simulink model "IP_LQR"  (R2020b)
settings: Solver=VariableStepAuto  StartTime=0.0  StopTime=5  RelTol=1e-3
values from neighbouring files (symbols this model uses):
  A = [0       1              0         0 ... (first row only)    [IP_Design.m]
  B = [     0 ... (first row only)    [IP_Design.m]
  C = [1 0 0 0 ... (first row only)    [IP_Design.m]
  D = zeros(2,1)    [IP_Design.m]
  K = lqr(A,B,Q,R)    [IP_Design.m]
  L = place(A',C',P)'    [IP_Design.m]
  m = 0.2    [Data_for_IP_Sim_Model.m]    (also in IP_Design.m)
  N = -1/(C*inv(Ac)*B)    [IP_Design.m]
  Qk = 0.005    [IP_Design.m]
  Rk = 0.001    [IP_Design.m]
  Sf = N(1,1)    [IP_Design.m]
undefined symbols (not defined in the file or in its folder): Continuous, sigbuilder_block, Time, X, Y, Z
libraries: sm_lib x8, nesl_utility x6, ctrlSharedLib x1
settings Model: Creator=tushark  LastModifiedBy=raghavendrans
settings ExplorerConfigSet: InternalSimMechanicsExplorerSettings="<ExplorerConfiguration><canonicalview>default</canonicalview><AnimationSetting><BasePlaybackSpeed>1.0</BasePlaybackSpeed><PlaybackSpeedFactor>1.0</PlaybackSpeedFactor></AnimationSetting><TilePanel><TileInfo><Tiles Columns=\"1\" Count=\"1\" Rows=\"1\"><Column Weight=\"1\"/><Row Weight=\"1\"/><Tile Height=\"1\" Width=\"1\" X=\"0\" Y=\"0\"/></Tiles></TileInfo><SceneInfo><SceneViewer><BGColor><R>1</R><G>1</G><B>1</B></BGColor><Camera><DoPerspective>off</DoPerspective><Position><X>0.288705906044352034</X><Y>-0.999999988114421923</Y><Z>0.250006416228108375</Z></Position><Center><X>0.288705906044352034</X><Y>1.18855781328086607e-08</Y><Z>0.250006416228108375</Z></Center><Up><X>0</X><Y>-0</Y><Z>1</Z></Up><ViewLimDist>1</ViewLimDist><YLim>0.360506624281406396</YLim><XLim>0.67276188393623837</XLim></Camera></SceneViewer></SceneInfo></TilePanel><MechEditorPanel><Cameras/><GfxPanelCameraMap/><VideoCreator><PlaybackSpeedRatio>1.0</PlaybackSpeedRatio><FrameRate>30</FrameRate><VideoFormat>Motion JPEG AVI</VideoFormat><FrameSize>auto</FrameSize></VideoCreator></MechEditorPanel></ExplorerConfiguration>"

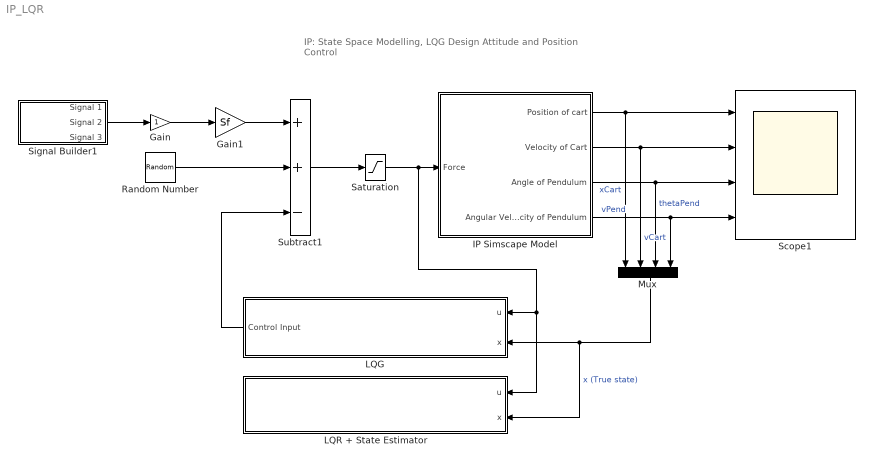
== system IP_LQR ==
  note: IP: State Space Modelling, LQG Design
      | Attitude and Position Control
  Gain : Gain
  Gain1 : Gain  Gain=Sf
  IP Simscape Model : Subsystem
  LQG : Subsystem
  LQR + State Estimator : Subsystem
  Mux : Mux
  Random Number : RandomNumber  Variance=Qk  SampleTime=0.1
  Saturation : Saturate  UpperLimit=1  LowerLimit=-1
  Scope1 : Scope  NumInputPorts=4
  Signal Builder1 : Subsystem  Tag=STV Subsys  LoadFcn=sigbuilder_block('load');  StartFcn=sigbuilder_block('start');  StopFcn=sigbuilder_block('stop');  ClipboardFcn=sigbuilder_block('clipboard');  mask(Sigbuilder block){tuvar=[0:10]}
      mask help: Simulink:masks:SigbuilderBlock_MD
      mask init:
      | if ~strcmp(get_param(bdroot(gcbh),'SimulationStatus'),'stopped') tuvar = sigbuilder_block('maskInit'); end
      settings: CopyFcn=sigbuilder_block('copy');  DeleteFcn=sigbuilder_block('delete');  ModelCloseFcn=sigbuilder_block('modelClose');  PreSaveFcn=sigbuilder_block('preSave');  PauseFcn=sigbuilder_block('pause');  ContinueFcn=sigbuilder_block('continue');  NameChangeFcn=sigbuilder_block('namechange');  OpenFcn=sigbuilder_block('open',[437.6 199.2 550.4 400 ]);  CloseFcn=sigbuilder_block('close');
      mask Display: plot(0, 0, 100, 100,[2, 2, 32, 32, 2], [68, 8, 8, 68, 68],[32, 2], [38, 38], [32, 19, 2],[53, 60, 44], [32, 17, 17, 2],[16, 16, 31, 31]);txt = getActiveGroup(gcbh);text(2, 100, txt,'verticalAlignment', 'top');
  Subtract1 : Sum  Inputs=++-
  wires:
  IP Simscape Model/1(Position of cart) -> Scope1/1, Mux/1  "xCart"
  IP Simscape Model/4(Angular Velocity of Pendulum) -> Scope1/4, Mux/4  "vPend"
  IP Simscape Model/3(Angle of Pendulum) -> Scope1/3, Mux/3  "thetaPend"
  IP Simscape Model/2(Velocity of Cart) -> Scope1/2, Mux/2  "vCart"
  Gain1/1 -> Subtract1/1
  Saturation/1 -> IP Simscape Model/1("Force "), LQR + State Estimator/1(u), LQG/1(u)
  Subtract1/1 -> Saturation/1
  Mux/1 -> LQR + State Estimator/2(x), LQG/2(x)  "x (True state)"
  Gain/1 -> Gain1/1
  Signal Builder1/2(Signal 2) -> Gain/1
  Random Number/1 -> Subtract1/2
  LQG/1("Control Input ") -> Subtract1/3

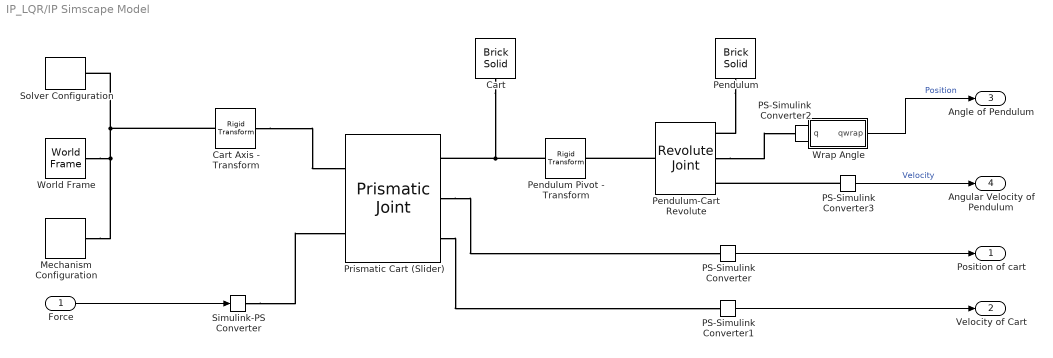
== system IP_LQR/IP Simscape Model ==
  "Force " : Inport
  Cart : sm_lib/Body Elements/Brick Solid  GraphicAmbientColor=[0.15 0.15 0.15 1.0]  BasedOnType=Density  BrickDimensions=[0.2 0.04 0.6]  BrickDimensionUnits=m  CenterOfMass=[0 0 0]  CenterOfMassUnits=m  GraphicDiffuseColor=[1.0 0.2 0.2]  Density=1000  DensityUnits=kg/m^3  DoExposeReferenceFrame=on  GraphicEmissiveColor=[0.0 0.0 0.0 1.0]  ExportEntireGeometry=off  SerializedFrames=<Frames/>  MarkerShape=Sphere  MarkerSize=10  GraphicType=FromGeometry  InertiaType=PointMass  Mass=0.5  MassUnits=kg  MomentsOfInertia=[1 1 1]  MomentsOfInertiaUnits=kg*m^2  GraphicOpacity=1.0  ProductsOfInertia=[0 0 0]  ProductsOfInertiaUnits=kg*m^2  GraphicShininess=75  GraphicSpecularColor=[0.5 0.5 0.5 1.0]  GraphicVisPropType=SimpleVisualProperties
  Cart Axis - Transform : sm_lib/Frames and Transforms/Rigid Transform  TranslationMethod=None  TranslationStandardOffset=0  TranslationLengthUnit=m  TranslationStandardAxis=+Z  TranslationCartesianOffset=[0 0 0]  TranslationROffset=0  TranslationROffsetUnits=m  TranslationZOffset=0  TranslationZOffsetUnits=m  TranslationThetaOffset=0  TranslationThetaOffsetUnits=deg  RotationMethod=StandardAxis  RotationAngleUnits=deg  RotationStandardAxis=+Y  RotationAngle=90  RotationArbitraryAxis=[0 0 1]  FollAlignAxisA=+X  BaseAlignAxisA=+Y  FollAlignAxisB=+Y  BaseAlignAxisB=+Z  RotationSequenceAxes=FollowerAxes  RotationSequence=XYX  RotationSequenceAngles=[0 0 0]  RotationSequenceAnglesUnits=deg  RotationMatrix=[1 0 0; 0 1 0; 0 0 1]
      settings: SourceProductName=Multibody
  Mechanism Configuration : sm_lib/Utilities/Mechanism Configuration  UniformGravity=Constant  GravityVector=[0 0 -9.80665]  GravityVectorUnits=m/s^2  GravityUnits=m/s^2  LinearizationDelta=0.001  JointModeTransitionNonlinearIterations=2
      settings: SourceProductName=Multibody
  PS-Simulink Converter{,1..3} (4 alike) : nesl_utility/PS-Simulink Converter  PhysicalDomain=network_engine_domain  SubClassName=ps_output  LeftPortType=input  RightPortType=output  PseudoPeriodic=off  Frequencies=[]  Unit=inherit  AffineConversion=off
  Pendulum : sm_lib/Body Elements/Brick Solid  GraphicAmbientColor=[0.15 0.15 0.15 1.0]  BasedOnType=Density  BrickDimensions=[0.6 0.03 0.05]  BrickDimensionUnits=m  CenterOfMass=[0 0 0]  CenterOfMassUnits=m  GraphicDiffuseColor=[0.0 0.4 1.0]  Density=1000  DensityUnits=kg/m^3  DoExposeReferenceFrame=off  GraphicEmissiveColor=[0.0 0.0 0.0 1.0]  ExportEntireGeometry=off  SerializedFrames=<Frames><Frame><Id>Frame1</Id><Value><Name>P</Name><Origin><Source>GeometricFeature</Source><FeatureName>+x surface</FeatureName></Origin><PrimaryAxis><DefinedDirection>+Z</DefinedDirection><Source>ReferenceFrame</Source><SourceDirection>+Z</SourceDirection><FeatureName></FeatureName></PrimaryAxis><SecondaryAxis><DefinedDirection>+X</DefinedDirection><Source>ReferenceFrame</Source><SourceDirection>+X</SourceDirection><FeatureName></FeatureName></SecondaryAxis></Value></Frame></Frames>  MarkerShape=Sphere  MarkerSize=10  GraphicType=FromGeometry  InertiaType=PointMass  Mass=0.2  MassUnits=kg  MomentsOfInertia=[1 1 1]  MomentsOfInertiaUnits=kg*m^2  GraphicOpacity=1.0  ProductsOfInertia=[0 0 0]  ProductsOfInertiaUnits=kg*m^2  GraphicShininess=75  GraphicSpecularColor=[0.5 0.5 0.5 1.0]  GraphicVisPropType=SimpleVisualProperties
  Pendulum Pivot - Transform : sm_lib/Frames and Transforms/Rigid Transform  TranslationMethod=None  TranslationStandardOffset=0  TranslationLengthUnit=m  TranslationStandardAxis=+Z  TranslationCartesianOffset=[0 0 0]  TranslationROffset=0  TranslationROffsetUnits=m  TranslationZOffset=0  TranslationZOffsetUnits=m  TranslationThetaOffset=0  TranslationThetaOffsetUnits=deg  RotationMethod=StandardAxis  RotationAngleUnits=deg  RotationStandardAxis=+X  RotationAngle=90  RotationArbitraryAxis=[0 0 1]  FollAlignAxisA=+X  BaseAlignAxisA=+Y  FollAlignAxisB=+Y  BaseAlignAxisB=+Z  RotationSequenceAxes=FollowerAxes  RotationSequence=XYX  RotationSequenceAngles=[0 0 0]  RotationSequenceAnglesUnits=deg  RotationMatrix=[1 0 0; 0 1 0; 0 0 1]
      settings: SourceProductName=Multibody
  Pendulum-Cart Revolute : sm_lib/Joints/Revolute Joint  JointMode=Normal  SenseConstraintForce=off  SenseConstraintForceX=off  SenseConstraintForceY=off  SenseConstraintForceZ=off  SenseConstraintTorque=off  SenseConstraintTorqueX=off  SenseConstraintTorqueY=off  SenseConstraintTorqueZ=off  SenseTotalForce=off  SenseTotalForceX=off  SenseTotalForceY=off  SenseTotalForceZ=off  SenseTotalTorque=off  SenseTotalTorqueX=off  SenseTotalTorqueY=off  SenseTotalTorqueZ=off  CompositeWrenchDir=FollowerOnBase  CompositeWrenchFrame=BaseFrame  EquilibriumPosition=0  EquilibriumPositionUnits=deg  SpringStiffness=0  SpringStiffnessUnits=N*m/deg  DampingCoefficient=0  DampingCoefficientUnits=N*m/(deg/s)  TorqueActuationMode=NoTorque  MotionActuationMode=ComputedMotion  SensePosition=on  SenseVelocity=on  SenseAcceleration=off  SenseTorqueForce=off  SenseLowerLimitTorqueForce=off  SenseUpperLimitTorqueForce=off  LowerLimitSpecify=off  LowerLimitBound=-90  LowerLimitBoundUnits=deg  LowerLimitStiffness=1e4  LowerLimitStiffnessUnits=N*m/deg  LowerLimitDamping=10  LowerLimitDampingUnits=N*m/(deg/s)  LowerLimitTransitionRegionWidth=0.1  LowerLimitTransitionRegionWidthUnits=deg  UpperLimitSpecify=off  UpperLimitBound=90  UpperLimitBoundUnits=deg  UpperLimitStiffness=1e4  UpperLimitStiffnessUnits=N*m/deg  UpperLimitDamping=10  UpperLimitDampingUnits=N*m/(deg/s)  UpperLimitTransitionRegionWidth=0.1  UpperLimitTransitionRegionWidthUnits=deg  PositionTargetSpecify=off  PositionTargetPriority=High  PositionTargetValue=0  PositionTargetValueUnits=deg  VelocityTargetSpecify=off  VelocityTargetPriority=High  VelocityTargetValue=0  VelocityTargetValueUnits=deg/s
  Prismatic Cart (Slider) : sm_lib/Joints/Prismatic Joint  JointMode=Normal  SenseConstraintForce=off  SenseConstraintForceX=off  SenseConstraintForceY=off  SenseConstraintForceZ=off  SenseConstraintTorque=off  SenseConstraintTorqueX=off  SenseConstraintTorqueY=off  SenseConstraintTorqueZ=off  SenseTotalForce=off  SenseTotalForceX=off  SenseTotalForceY=off  SenseTotalForceZ=off  SenseTotalTorque=off  SenseTotalTorqueX=off  SenseTotalTorqueY=off  SenseTotalTorqueZ=off  CompositeWrenchDir=FollowerOnBase  CompositeWrenchFrame=BaseFrame  EquilibriumPosition=0  EquilibriumPositionUnits=m  SpringStiffness=0  SpringStiffnessUnits=N/m  DampingCoefficient=0.1  DampingCoefficientUnits=N/(m/s)  TorqueActuationMode=InputTorque  MotionActuationMode=ComputedMotion  SensePosition=on  SenseVelocity=on  SenseAcceleration=off  SenseTorqueForce=off  SenseLowerLimitTorqueForce=off  SenseUpperLimitTorqueForce=off  LowerLimitSpecify=on  LowerLimitBound=-1  LowerLimitBoundUnits=m  LowerLimitStiffness=1e6  LowerLimitStiffnessUnits=N/m  LowerLimitDamping=1e3  LowerLimitDampingUnits=N/(m/s)  LowerLimitTransitionRegionWidth=1e-4  LowerLimitTransitionRegionWidthUnits=m  UpperLimitSpecify=on  UpperLimitBound=1  UpperLimitBoundUnits=m  UpperLimitStiffness=1e6  UpperLimitStiffnessUnits=N/m  UpperLimitDamping=1e3  UpperLimitDampingUnits=N/(m/s)  UpperLimitTransitionRegionWidth=1e-4  UpperLimitTransitionRegionWidthUnits=m  PositionTargetSpecify=off  PositionTargetPriority=High  PositionTargetValue=0  PositionTargetValueUnits=m  VelocityTargetSpecify=off  VelocityTargetPriority=High  VelocityTargetValue=0  VelocityTargetValueUnits=m/s
  Simulink-PS Converter : nesl_utility/Simulink-PS Converter  PhysicalDomain=network_engine_domain  SubClassName=ps_input  LeftPortType=input  RightPortType=output  PseudoPeriodic=off  Frequencies=[]  NoiseDistribution=none  NoiseParameters=[]  Unit=1  AffineConversion=off  FilteringAndDerivatives=provide  SimscapeFilterOrder=1  InputFilterTimeConstant=0.001  UdotUserProvided=0
  Solver Configuration : nesl_utility/Solver Configuration  PhysicalDomain=network_engine_domain  SubClassName=solver  LeftPortType=input  RightPortType=generic  Tones=[]  Harmonics=[]  SimulateNoise=off  Profile=off  UseLocalSampling=off  EnableSwitchedLinearOptims=on  FrequencyDomain=off  UseCCode=off  RelTol=0.001  AbsTol=1e-06  MinStep=1e-09  ToWorkspace=off  RevertToSquareIcSolve=off  NumHomotopyIterations=100  PhasorMode=off  PhasorModeNumHarmonics=1  DoDC=off  ResidualTolerance=1e-09  UseLocalSolver=off  LocalSolverChoice=NE_BACKWARD_EULER_ADVANCER  LocalSolverSampleTime=0.001  DoFixedCost=off  MaxNonlinIter=3  MaxModeIter=2  ComputeImpulses=off  ImpulseIterations=2  LinearAlgebra=Sparse  EquationFormulation=NE_TIME_EF  DelaysMemoryBudget=1024  AutomaticFiltering=on  FilteringTimeConstant=0.001  PartitionStorageMethod=AS_NEEDED  PartitionMemoryBudget=1024  PartitionMethod=FAST
      settings: SourceProductName=Utilities
  World Frame : sm_lib/Frames and Transforms/World Frame
      settings: SourceProductName=Multibody
  Wrap Angle : Subsystem
  Position of cart : Outport
  Velocity of Cart : Outport  Port=2
  Angle of Pendulum : Outport  Port=3
  Angular Velocity of Pendulum : Outport  Port=4
  wires:
  PS-Simulink Converter1/1 -> Velocity of Cart/1
  PS-Simulink Converter/1 -> Position of cart/1
  Wrap Angle/1(qwrap) -> Angle of Pendulum/1  "Position"
  "Force "/1 -> Simulink-PS Converter/1
  PS-Simulink Converter2/1 -> Wrap Angle/1(q)
  PS-Simulink Converter3/1 -> Angular Velocity of Pendulum/1  "Velocity"
  connections:
  Prismatic Cart (Slider)/RConn3 -- PS-Simulink Converter1/LConn1
  Prismatic Cart (Slider)/RConn2 -- PS-Simulink Converter/LConn1
  Cart/RConn1 -- Prismatic Cart (Slider)/RConn1 -- Pendulum Pivot - Transform/LConn1
  PS-Simulink Converter3/LConn1 -- Pendulum-Cart Revolute/RConn3
  World Frame/RConn1 -- Cart Axis - Transform/LConn1 -- Solver Configuration/RConn1 -- Mechanism Configuration/RConn1
  Cart Axis - Transform/RConn1 -- Prismatic Cart (Slider)/LConn1
  Pendulum-Cart Revolute/RConn2 -- PS-Simulink Converter2/LConn1
  Pendulum-Cart Revolute/LConn1 -- Pendulum Pivot - Transform/RConn1
  Simulink-PS Converter/RConn1 -- Prismatic Cart (Slider)/LConn2
  Pendulum/LConn1 -- Pendulum-Cart Revolute/RConn1

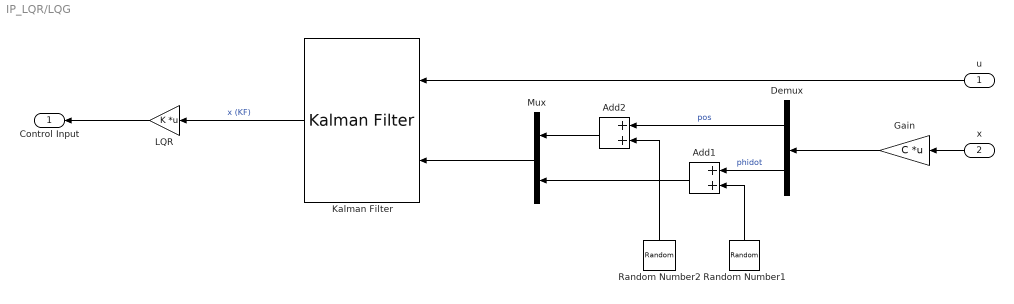
== system IP_LQR/LQG ==
  u : Inport
  x : Inport  Port=2
  "    LQR " : Gain  Gain=K  Multiplication=Matrix(K*u)
  Add1 : Sum
  Add2 : Sum
  Demux : Demux  Outputs=2
  Gain : Gain  Gain=C  Multiplication=Matrix(K*u) (u vector)
  Kalman Filter : ctrlSharedLib/Kalman Filter  TimeDomain=Continuous-Time  UseCurrentEstimator=on  ModelSource=Individual A, B, C, D matrices  ModelSourceVariable=ss(0.95,1,1,0,1)  A=A  B=B  C=C  D=D  NumberOfStates=1  NumberOfInputs=1  NumberOfOutputs=1  InitialEstimateSource=Dialog  X0=0  P0=10  UseK=off  UseGH=off  NumberOfProcessNoiseInputs=1  G=1  TimeInvariantG=on  H=0  TimeInvariantH=on  Q=Qk.*eye(4)  TimeInvariantQ=on  R=Rk.*eye(2)  TimeInvariantR=on  N=0  TimeInvariantN=on  AddInputPort=on  AddEnablePort=off  OutputEstimatedY=off  OutputP=off  Ts=-1
  Mux : Mux  Inputs=2
  Random Number1 : RandomNumber  Variance=Rk
  Random Number2 : RandomNumber  Variance=Rk
  "Control Input " : Outport
  wires:
  "    LQR "/1 -> "Control Input "/1
  u/1 -> Kalman Filter/1
  Kalman Filter/1 -> "    LQR "/1  "x (KF)"
  x/1 -> Gain/1
  Mux/1 -> Kalman Filter/2
  Gain/1 -> Demux/1
  Demux/1 -> Add2/1  "pos"
  Demux/2 -> Add1/1  "phidot"
  Random Number1/1 -> Add1/2
  Random Number2/1 -> Add2/2
  Add1/1 -> Mux/2
  Add2/1 -> Mux/1

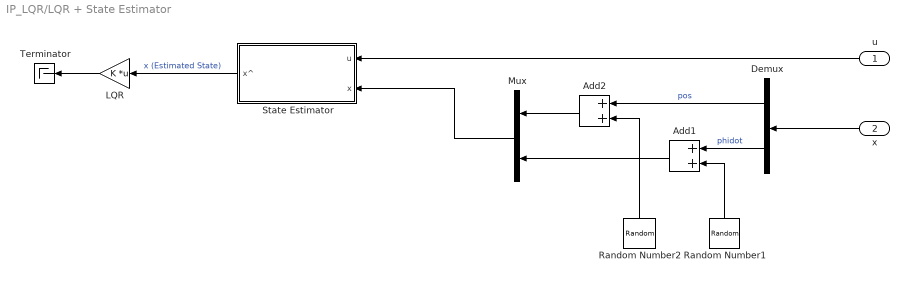
== system IP_LQR/LQR + State Estimator ==
  u : Inport
  x : Inport  Port=2
  "   LQR" : Gain  Gain=K  Multiplication=Matrix(K*u)
  Add1 : Sum
  Add2 : Sum
  Demux : Demux  Outputs=2
  Mux : Mux  Inputs=2
  Random Number1 : RandomNumber  Variance=Rk
  Random Number2 : RandomNumber  Variance=Rk
  State Estimator : Subsystem
  Terminator : Terminator
  wires:
  u/1 -> State Estimator/1(u)
  State Estimator/1(x^) -> "   LQR"/1  "x (Estimated State)"
  Add1/1 -> Mux/2
  Random Number1/1 -> Add1/2
  Add2/1 -> Mux/1
  x/1 -> Demux/1
  Mux/1 -> State Estimator/2(x)
  Demux/2 -> Add1/1  "phidot"
  Random Number2/1 -> Add2/2
  Demux/1 -> Add2/1  "pos"
  "   LQR"/1 -> Terminator/1

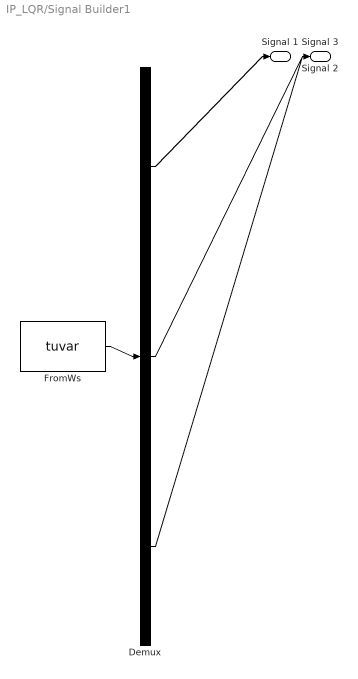
== system IP_LQR/Signal Builder1 ==
  Demux : Demux  Tag=STV Demux  Outputs=3
      settings: DisplayOption=none
  FromWs : FromWorkspace  Tag=STV FromWs  VariableName=tuvar
      SigBuilderData=|
      | common.afterFinalStr = 'Extrapolate'
      | common.sampleTime = 0
      | dataSet.timeRange = [0 10]
      | dataSet.name = 'Group 1'
      | sbobj.Groups.Name = 'Group 1'
      | sbobj.Groups.Signals(1).Name = 'Signal 1'
      | sbobj.Groups.Signals(1).XData = [0 10]
      | sbobj.Groups.Signals(1).YData = [0.3 0.3]
      | sbobj.Groups.Signals(2).Name = 'Signal 2'
      | sbobj.Groups.Signals(2).XData = [0 1 1 10]
      | sbobj.Groups.Signals(2).YData = [0.3 0.3 0 0]
      | sbobj.Groups.Signals(3).Name = 'Signal 3'
      | sbobj.Groups.Signals(3).XData = [0 1 1 10]
      | sbobj.Groups.Signals(3).YData = [0 0 0.3 0.3]
  Signal 1 : Outport  Tag=STV Outport
  Signal 2 : Outport  Tag=STV Outport  Port=2
  Signal 3 : Outport  Tag=STV Outport  Port=3
  wires:
  Demux/1 -> Signal 1/1
  Demux/2 -> Signal 2/1
  Demux/3 -> Signal 3/1
  FromWs/1 -> Demux/1

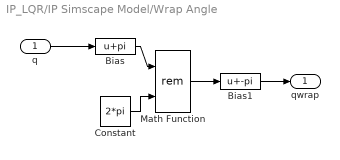
== system IP_LQR/IP Simscape Model/Wrap Angle ==
  q : Inport
  Bias : Bias  Bias=pi
  Bias1 : Bias  Bias=-pi
  Constant : Constant  Value=2*pi
  Math Function : Math  Operator=rem  SignedPower=on  SaturateOnIntegerOverflow=on
  qwrap : Outport  VectorParamsAs1DForOutWhenUnconnected=off
  wires:
  q/1 -> Bias/1
  Constant/1 -> Math Function/2
  Math Function/1 -> Bias1/1
  Bias/1 -> Math Function/1
  Bias1/1 -> qwrap/1

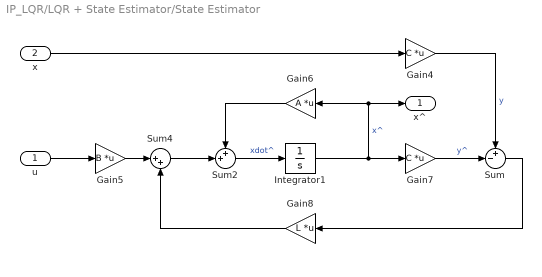
== system IP_LQR/LQR + State Estimator/State Estimator ==
  u : Inport
  x : Inport  Port=2
  Gain4 : Gain  Gain=C  Multiplication=Matrix(K*u)
  Gain5 : Gain  Gain=B  Multiplication=Matrix(K*u)
  Gain6 : Gain  Gain=A  Multiplication=Matrix(K*u)
  Gain7 : Gain  Gain=C  Multiplication=Matrix(K*u)
  Gain8 : Gain  Gain=L  Multiplication=Matrix(K*u)
  Integrator1 : Integrator
  Sum : Sum  Inputs=+-|
  Sum2 : Sum  Inputs=++|
  Sum4 : Sum  Inputs=|++
  x^ : Outport
  wires:
  Gain4/1 -> Sum/1  "y"
  Sum2/1 -> Integrator1/1  "xdot^"
  Gain8/1 -> Sum4/2
  Gain6/1 -> Sum2/1
  Sum/1 -> Gain8/1
  Gain7/1 -> Sum/2  "y^"
  Integrator1/1 -> Gain6/1, x^/1, Gain7/1  "x^"
  x/1 -> Gain4/1
  u/1 -> Gain5/1
  Gain5/1 -> Sum4/1
  Sum4/1 -> Sum2/2
